simulink library "waijung_input_validation"  (Simulink 7.3)
settings: Solver=ode45  StartTime=0.0  StopTime=10.0  RelTol=1e-3
libraries: simulink x9
settings Model: Creator=Krisada  LastModifiedBy=Krisada

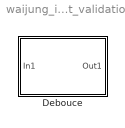
== system waijung_input_validation ==
  Debouce : Subsystem  TreatAsAtomicUnit=on  mask{mode=Normal, prescale=4, debouce=3}
      mask prompts: prescale "Prescale (Debouce count)"; debouce "Debouce value"
      settings: RTWFcnNameOpts=Use subsystem name  RTWFileNameOpts=Use function name
      mask StyleString: popup(Normal|Single Pulse|Toggle Latch),popup(4|8|16|32|64|128|256|512|1024|2048|4096|8192),edit
      mask CallbackString: waijung_intput_validation_callback('mode');||waijung_intput_validation_callback('prescale');
      mask Display: disp('Button Pressed\n(Normal)');

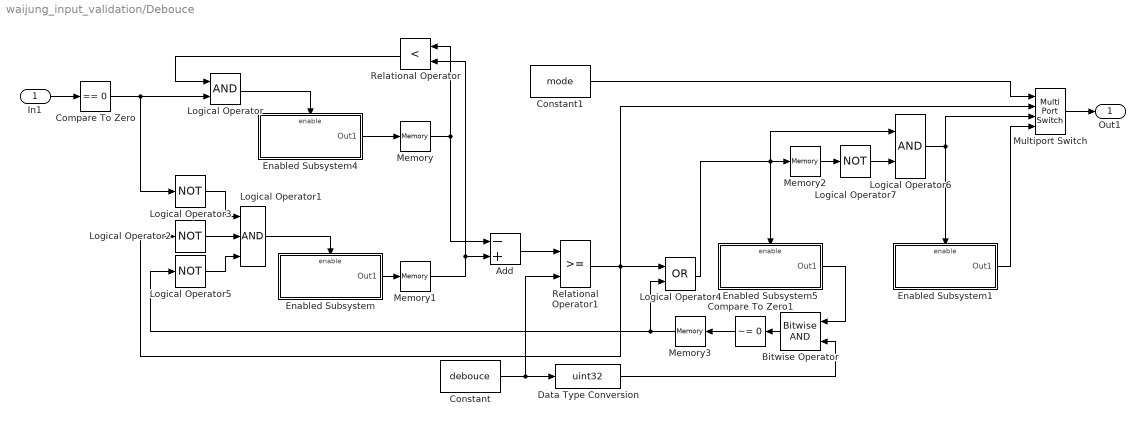
== system waijung_input_validation/Debouce ==
  In1 : Inport  OutDataType=fixdt(1, 16)  OutScaling=2^0
  Add : Sum  Inputs=-+  OutDataTypeMode=int32  OutDataType=fixdt(1, 16)  OutScaling=2^-10  OutDataTypeStr=int32
  Bitwise Operator : simulink/Logic and Bit Operations/Bitwise Operator  logicop=AND  UseBitMask=off  NumInputPorts=2  BitMask=debouce  BitMaskRealWorld=Stored Integer
  Compare To Zero : simulink/Logic and Bit Operations/Compare To Zero  SystemSampleTime=-1  relop===  LogicOutDataTypeMode=uint8  ZeroCross=off
  Compare To Zero1 : simulink/Logic and Bit Operations/Compare To Zero  SystemSampleTime=-1  relop=~=  LogicOutDataTypeMode=boolean  ZeroCross=off
  Constant : Constant  Value=debouce  OutDataTypeMode=int32  OutDataType=fixdt(1, 16)  OutScaling=2^0  OutDataTypeStr=int32
  Constant1 : Constant  Value=mode  OutDataTypeMode=int32  OutDataType=fixdt(1, 16)  OutScaling=2^0  OutDataTypeStr=int32
  Data Type Conversion : DataTypeConversion  OutDataTypeMode=uint32  OutDataType=fixdt(1, 16)  OutScaling=2^0  OutDataTypeStr=uint32
  Enabled Subsystem : Subsystem  TreatAsAtomicUnit=on
  Enabled Subsystem1 : Subsystem  TreatAsAtomicUnit=on
  Enabled Subsystem4 : Subsystem  TreatAsAtomicUnit=on
  Enabled Subsystem5 : Subsystem  TreatAsAtomicUnit=on
  Logical Operator : Logic  AllPortsSameDT=off  OutDataTypeMode=boolean  LogicDataType=fixdt(0, 8)  OutDataTypeStr=boolean
  Logical Operator1 : Logic  Inputs=3  AllPortsSameDT=off  OutDataTypeMode=boolean  LogicDataType=fixdt(0, 8)  OutDataTypeStr=boolean
  Logical Operator{2..3,5,7} (4 alike) : Logic  Operator=NOT  AllPortsSameDT=off  OutDataTypeMode=boolean  LogicDataType=fixdt(0, 8)  OutDataTypeStr=boolean
  Logical Operator4 : Logic  Operator=OR  AllPortsSameDT=off  OutDataTypeMode=boolean  LogicDataType=fixdt(0, 8)  OutDataTypeStr=boolean
  Logical Operator6 : Logic  AllPortsSameDT=off  OutDataTypeMode=boolean  LogicDataType=fixdt(0, 8)  OutDataTypeStr=boolean
  Memory{,1..3} (4 alike) : Memory  LinearizeMemory=on
  Multiport Switch : MultiPortSwitch  OutDataType=fixdt(1, 16)  OutScaling=2^0
  Relational Operator : RelationalOperator  Operator=<  LogicOutDataTypeMode=boolean  LogicDataType=fixdt(0, 8)  OutDataTypeStr=boolean
  Relational Operator1 : RelationalOperator  LogicOutDataTypeMode=boolean  LogicDataType=fixdt(0, 8)  OutDataTypeStr=boolean  InputSameDT=on
  Out1 : Outport  OutDataType=fixdt(1, 16)  OutScaling=2^0
  wires:
  Logical Operator1/1 -> Enabled Subsystem/Enable
  Relational Operator1/1 -> Logical Operator2/1, Logical Operator4/1, Multiport Switch/2
  Logical Operator7/1 -> Logical Operator6/2
  Memory2/1 -> Logical Operator7/1
  Logical Operator4/1 -> Logical Operator6/1, Memory2/1, Enabled Subsystem5/Enable
  Enabled Subsystem5/1(Out1) -> Bitwise Operator/1
  Bitwise Operator/1 -> Compare To Zero1/1
  Compare To Zero1/1 -> Memory3/1
  Logical Operator3/1 -> Logical Operator1/1
  Logical Operator5/1 -> Logical Operator1/3
  Memory3/1 -> Logical Operator5/1, Logical Operator4/2
  Logical Operator2/1 -> Logical Operator1/2
  Constant/1 -> Relational Operator1/2, Data Type Conversion/1
  Add/1 -> Relational Operator1/1
  Relational Operator/1 -> Logical Operator/1
  Logical Operator/1 -> Enabled Subsystem4/Enable
  Compare To Zero/1 -> Logical Operator3/1, Logical Operator/2
  Memory1/1 -> Relational Operator/2, Add/2
  Memory/1 -> Add/1, Relational Operator/1
  Enabled Subsystem4/1(Out1) -> Memory/1
  Enabled Subsystem/1(Out1) -> Memory1/1
  In1/1 -> Compare To Zero/1
  Logical Operator6/1 -> Multiport Switch/3, Enabled Subsystem1/Enable
  Enabled Subsystem1/1(Out1) -> Multiport Switch/4
  Data Type Conversion/1 -> Bitwise Operator/2
  Multiport Switch/1 -> Out1/1
  Constant1/1 -> Multiport Switch/1

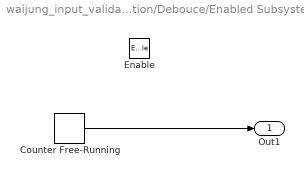
== system waijung_input_validation/Debouce/Enabled Subsystem ==
  Enable : EnablePort
  Counter Free-Running : simulink/Sources/Counter Free-Running  SystemSampleTime=-1  NumBits=32  tsamp=-1
  Out1 : Outport  OutDataType=fixdt(1, 16)  OutScaling=2^0  InitialOutput=0
  wires:
  Counter Free-Running/1 -> Out1/1

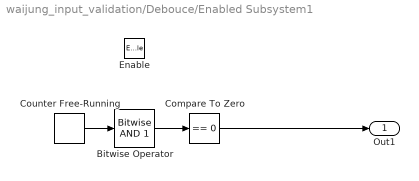
== system waijung_input_validation/Debouce/Enabled Subsystem1 ==
  Enable : EnablePort
  Bitwise Operator : simulink/Logic and Bit Operations/Bitwise Operator  logicop=AND  UseBitMask=on  BitMask=1  BitMaskRealWorld=Stored Integer
  Compare To Zero : simulink/Logic and Bit Operations/Compare To Zero  SystemSampleTime=-1  relop===  LogicOutDataTypeMode=uint8  ZeroCross=off
  Counter Free-Running : simulink/Sources/Counter Free-Running  SystemSampleTime=-1  NumBits=32  tsamp=-1
  Out1 : Outport  OutDataType=fixdt(1, 16)  OutScaling=2^0  InitialOutput=0
  wires:
  Compare To Zero/1 -> Out1/1
  Bitwise Operator/1 -> Compare To Zero/1
  Counter Free-Running/1 -> Bitwise Operator/1

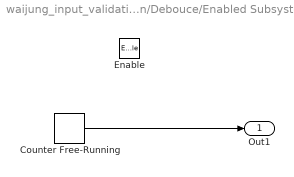
== system waijung_input_validation/Debouce/Enabled Subsystem4 ==
  Enable : EnablePort
  Counter Free-Running : simulink/Sources/Counter Free-Running  SystemSampleTime=-1  NumBits=32  tsamp=-1
  Out1 : Outport  OutDataType=fixdt(1, 16)  OutScaling=2^0  InitialOutput=0
  wires:
  Counter Free-Running/1 -> Out1/1

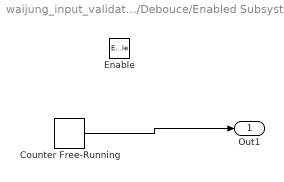
== system waijung_input_validation/Debouce/Enabled Subsystem5 ==
  Enable : EnablePort
  Counter Free-Running : simulink/Sources/Counter Free-Running  SystemSampleTime=-1  NumBits=32  tsamp=-1
  Out1 : Outport  OutDataType=fixdt(1, 16)  OutScaling=2^0  InitialOutput=0
  wires:
  Counter Free-Running/1 -> Out1/1
